simulink model "TP2_varying_antigo"  (R2020a)
settings: Solver=VariableStepAuto  StartTime=0.0  StopTime=10.0  RelTol=1e-3
values from neighbouring files (symbols this model uses):
  K = place(A,B,p)    [TP2.m]
undefined symbols (not defined in the file or in its folder): A, B, C, DiscIntNeverNeededParam, posicao, velocidade
libraries: cstblocks x2
settings Model: Creator=João  LastModifiedBy=João
settings DebuggingCC: UnderSpecifiedDimensionMsg=warning

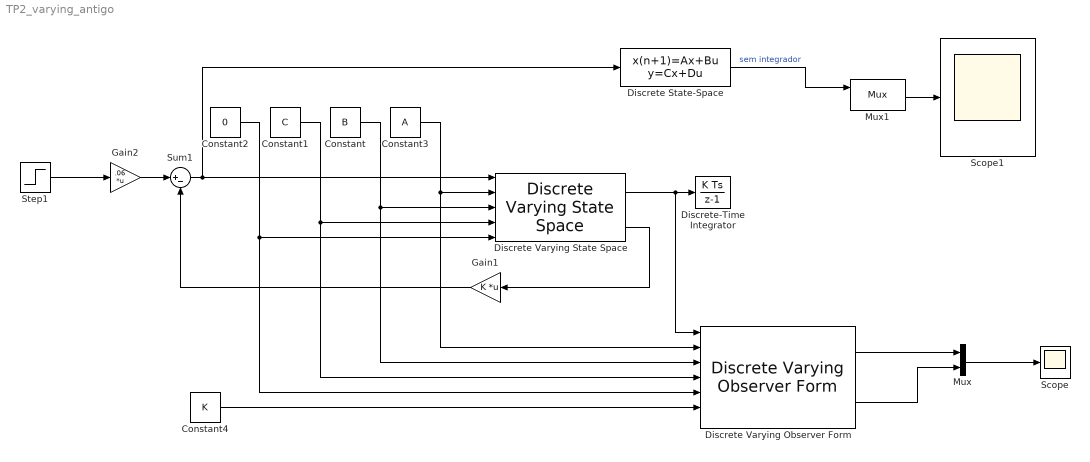
== system TP2_varying_antigo ==
  Constant : Constant  Value=B  VectorParams1D=off  SampleTime=-1
  Constant1 : Constant  Value=C  VectorParams1D=off  SampleTime=-1
  Constant2 : Constant  Value=0  VectorParams1D=off  SampleTime=-1
  Constant3 : Constant  Value=A  VectorParams1D=off  SampleTime=-1
  Constant4 : Constant  Value=K  VectorParams1D=off
  Discrete State-Space : DiscreteStateSpace  A=A  B=B  C=C  D=0  SampleTime=-1  StateName=[posicao velocidade]
  Discrete Varying Observer Form : cstblocks/Linear Parameter Varying/Discrete Varying Observer Form  x0=0  Ts=-1  OutputX=on  OutputDX=off
      settings: SourceProductBaseCode=CT
  Discrete Varying State Space : cstblocks/Linear Parameter Varying/Discrete Varying State Space  x0=0  Ts=-1  OutputX=on  OutputDX=off
      settings: SourceProductBaseCode=CT
  Discrete-Time Integrator : DiscreteIntegrator  gainval=5  SampleTime=-1  ICPrevOutput=DiscIntNeverNeededParam  ICPrevScaledInput=DiscIntNeverNeededParam
  Gain1 : Gain  Gain=K  Multiplication=Matrix(K*u) (u vector)
  Gain2 : Gain  Gain=.06  Multiplication=Matrix(K*u)
  Mux : Mux  Inputs=2
  Mux1 : Mux  Inputs=2
      settings: DisplayOption=signals
  Scope : Scope
  Scope1 : Scope
  Step1 : Step  After=10  SampleTime=0
  Sum1 : Sum  Inputs=|+-
  wires:
  Discrete Varying State Space/2 -> Gain1/1
  Gain1/1 -> Sum1/2
  Sum1/1 -> Discrete Varying State Space/1, Discrete State-Space/1
  Constant3/1 -> Discrete Varying Observer Form/2, Discrete Varying State Space/2
  Constant2/1 -> Discrete Varying Observer Form/5, Discrete Varying State Space/5
  Constant1/1 -> Discrete Varying Observer Form/4, Discrete Varying State Space/4
  Constant/1 -> Discrete Varying Observer Form/3, Discrete Varying State Space/3
  Discrete Varying State Space/1 -> Discrete-Time Integrator/1, Discrete Varying Observer Form/1
  Constant4/1 -> Discrete Varying Observer Form/6
  Mux/1 -> Scope/1
  Step1/1 -> Gain2/1
  Gain2/1 -> Sum1/1
  Mux1/1 -> Scope1/1
  Discrete Varying Observer Form/1 -> Mux/1
  Discrete Varying Observer Form/2 -> Mux/2
  Discrete State-Space/1 -> Mux1/1  "sem integrador"
